simulink model "ePowertrain model"  (R2024b)
settings: Solver=VariableStepAuto  StartTime=0.0  StopTime=time  RelTol=1e-3
model workspace (MATLAB code in the model file):
  | RW = 0.254 ; % radius of vehicle (m)
  | GVM = 330 ; % gross vehicle mass (kg)
  | GVW = GVM*9.81 ; % gross vehicle weight (kg.m/s^2)
  | Crf = 0.015 ; % coeff of rolling resistance
  | slope_angle = 0 ; %slope angle in radian
  | Af = 1.1 ; %frontal Area (m^2)
  | Cd = 0.4 ; % coeff of drag
  | gear_ratio = 6 ;
  | trans_eff = 0.9; % transmission efficiency
  | motor_eff = 0.9; % motor efficiency
  | mc_eff = 0.95; % motor controller efficiency
  | Bv = 72 ; % battery voltage (V)
  | Cv = 3.6 ; % nominated cell votage (V)
  | Cc = 31 ; % cell capacity (Ah)
  | 
  | lap_distance = 0.787 ; % distance of one lap (km)
  | range = 20; % range of vehicle in single charge
  | time = 60 ; % time required to complete one lap
  | air_density = 1.225 ;
settings Model: Creator=chikr  LastModifiedBy=chikr

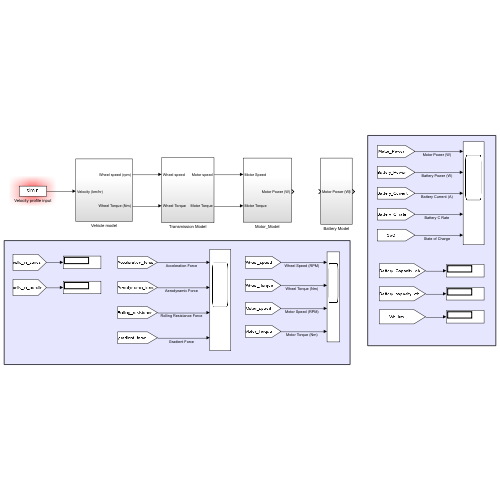
[thumbnail: Simulink's stored preview of the top-level diagram]
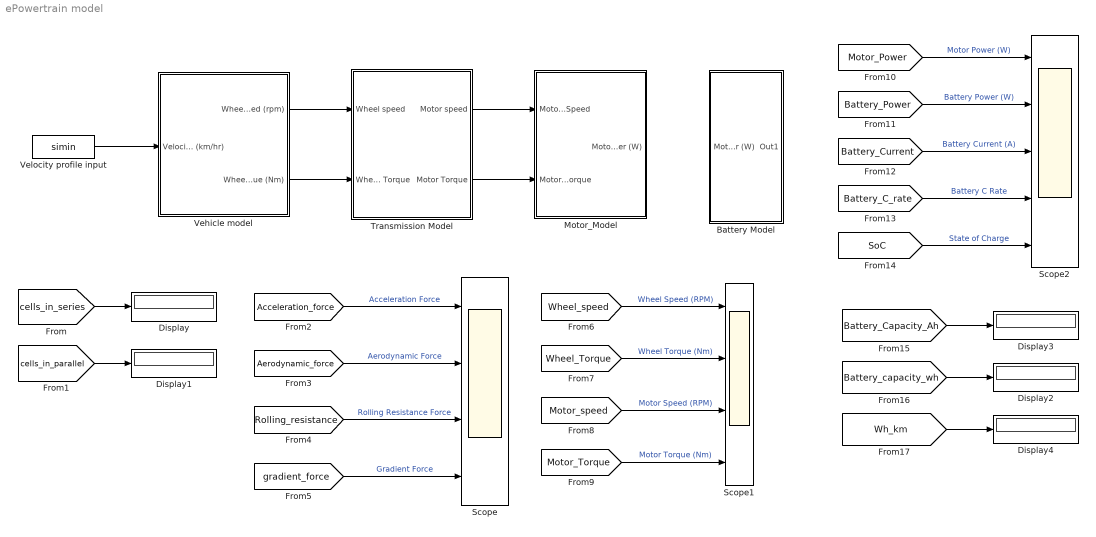
== system ePowertrain model ==
  Battery Model : Subsystem
  Display{,1..4} (5 alike) : Display
  Motor_Model : Subsystem
  Scope : Scope  NumInputPorts=4
  Scope1 : Scope  NumInputPorts=4
  Scope2 : Scope  NumInputPorts=5
  Transmission Model : Subsystem
  Vehicle model : Subsystem
  Velocity profile input : FromWorkspace  VariableName=simin
  wires:
  Velocity profile input/1 -> Vehicle model/1(Velocity (km/hr))
  Vehicle model/2(Wheel Torque (Nm)) -> Transmission Model/2(Wheel Torque)
  Vehicle model/1(Wheel speed (rpm)) -> Transmission Model/1(Wheel speed)
  Transmission Model/2(Motor Torque) -> Motor_Model/2(Motor Torque)
  Transmission Model/1(Motor speed) -> Motor_Model/1(Motor Speed)
  [cells_in_series] -> Display/1
  [cells_in_parallel] -> Display1/1
  [Acceleration_force] -> Scope/1  "Acceleration Force"
  [Aerodynamic_force] -> Scope/2  "Aerodynamic Force"
  [Rolling_resistance] -> Scope/3  "Rolling Resistance Force"
  [gradient_force] -> Scope/4  "Gradient Force"
  [Wheel_speed] -> Scope1/1  "Wheel Speed (RPM)"
  [Wheel_Torque] -> Scope1/2  "Wheel Torque (Nm)"
  [Motor_speed] -> Scope1/3  "Motor Speed (RPM)"
  [Motor_Torque] -> Scope1/4  "Motor Torque (Nm)"
  [Motor_Power] -> Scope2/1  "Motor Power (W)"
  [Battery_Current] -> Scope2/3  "Battery Current (A)"
  [Battery_Power] -> Scope2/2  "Battery Power (W)"
  [Battery_C_rate] -> Scope2/4  "Battery C Rate"
  [SoC] -> Scope2/5  "State of Charge"
  [Wh_km] -> Display4/1
  [Battery_capacity_wh] -> Display2/1
  [Battery_Capacity_Ah] -> Display3/1

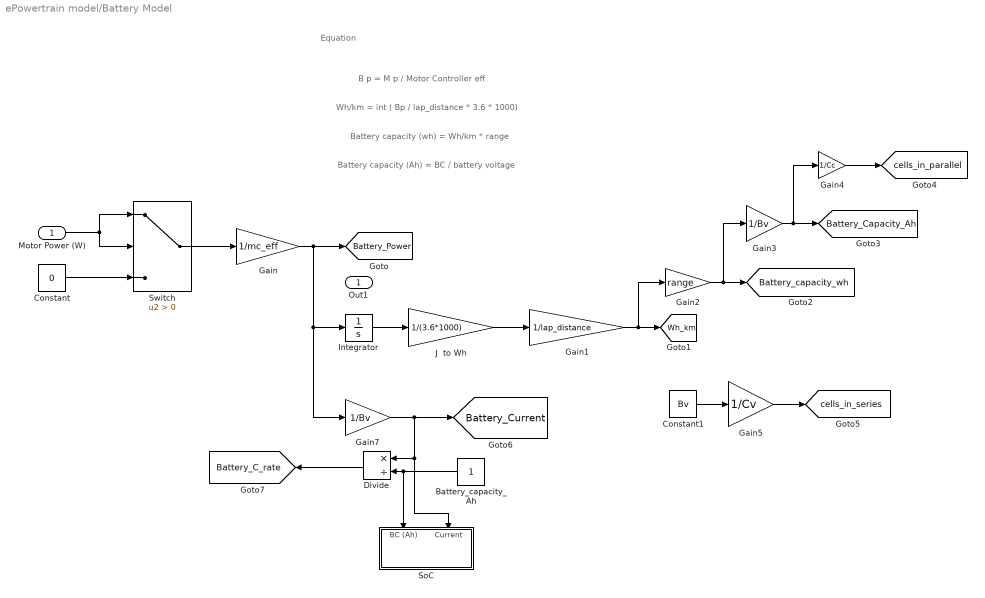
== system ePowertrain model/Battery Model ==
  note: Battery capacity (Ah) = BC / battery voltage
  note: Battery capacity (wh) = Wh/km * range
  note: Wh/km = int ( Bp / lap_distance * 3.6 * 1000)
  note: Equation
  note: B p = M p / Motor Controller eff
  Motor Power (W) : Inport
  Battery_capacity_Ah : Constant
  Constant : Constant  Value=0
  Constant1 : Constant  Value=Bv
  Divide : Product  Inputs=*/
  Gain : Gain  Gain=1/mc_eff
  Gain1 : Gain  Gain=1/lap_distance
  Gain2 : Gain  Gain=range
  Gain3 : Gain  Gain=1/Bv
  Gain4 : Gain  Gain=1/Cc
  Gain5 : Gain  Gain=1/Cv
  Gain7 : Gain  Gain=1/Bv
  Integrator : Integrator
  J  to Wh : Gain  Gain=1/(3.6*1000)
  SoC : Subsystem
      settings: PortSchema="{\"entries\":[{\"content\":{\"sides\":[{\"content\":{},\"type\":\"ConnectorPlacement.EquallySpacedRectSide\",\"uuid\":\"75e15061-75ea-40ab-85e0-9adabe2f895d\"},{\"content\":{\"side\":\"RIGHT\"},\"type\":\"ConnectorPlacement.EquallySpacedRectSide\",\"uuid\":\"53768e5b-e8ce-4d09-bbe5-28fa4e20151a\"},{\"content\":{\"connectorIds\":[\"In1\",\"In2\"],\"side\":\"TOP\"},\"type\":\"ConnectorPlacement.EquallySpacedRectSide\",\"uuid\":\"7db4e560-ff94-4941-b244-cacdfd66e211\"}]},\"type\":\"ConnectorPlacement.EquallySpacedConnector\",\"uuid\":\"b200b510-6a7e-48d6-8933-7bee46b324cd\"}],\"packageUris\":[\"http://schema.mathworks.com/mf0/Connector/R2020b\"],\"version\":\"1.0\"}"
  Switch : Switch  Criteria=u2 > Threshold  SaturateOnIntegerOverflow=off  InputSameDT=off
  Out1 : Outport
  tag scope: Battery_C_rate=global, Battery_Capacity_Ah=global, Battery_Current=global, Battery_Power=global, Battery_capacity_wh=global, Wh_km=global, cells_in_parallel=global, cells_in_series=global
  wires:
  Motor Power (W)/1 -> Switch/2, Switch/1
  Constant/1 -> Switch/3
  Switch/1 -> Gain/1
  Gain/1 -> Gain7/1, Integrator/1, [Battery_Power]
  Integrator/1 -> J  to Wh/1
  J  to Wh/1 -> Gain1/1
  Gain1/1 -> Gain2/1, [Wh_km]
  Gain2/1 -> Gain3/1, [Battery_capacity_wh]
  Gain3/1 -> Gain4/1, [Battery_Capacity_Ah]
  Gain4/1 -> [cells_in_parallel]
  Constant1/1 -> Gain5/1
  Gain5/1 -> [cells_in_series]
  Gain7/1 -> [Battery_Current], SoC/2(Current), Divide/1
  Battery_capacity_Ah/1 -> SoC/1(BC (Ah)), Divide/2
  Divide/1 -> [Battery_C_rate]

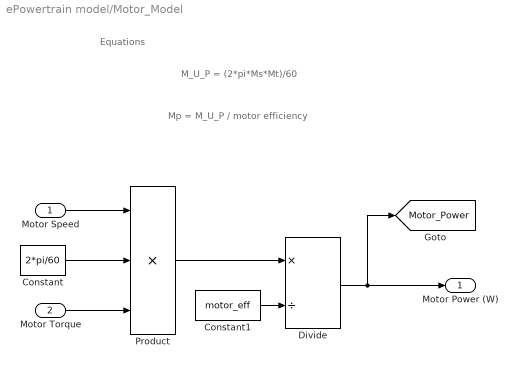
== system ePowertrain model/Motor_Model ==
  note: Equations
  note: Mp = M_U_P / motor efficiency
  note: M_U_P = (2*pi*Ms*Mt)/60
  Motor Speed : Inport
  Motor Torque : Inport  Port=2
  Constant : Constant  Value=2*pi/60
  Constant1 : Constant  Value=motor_eff
  Divide : Product  Inputs=*/
  Product : Product  Inputs=3
  Motor Power (W) : Outport
  tag scope: Motor_Power=global
  wires:
  Motor Speed/1 -> Product/1
  Motor Torque/1 -> Product/3
  Constant/1 -> Product/2
  Product/1 -> Divide/1
  Constant1/1 -> Divide/2
  Divide/1 -> [Motor_Power], Motor Power (W)/1

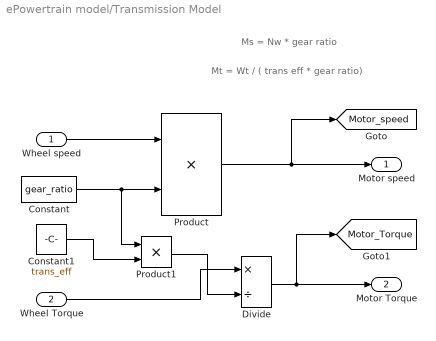
== system ePowertrain model/Transmission Model ==
  note: Mt = Wt / ( trans eff * gear ratio)
  note: Ms = Nw * gear ratio
  Wheel speed : Inport
  Wheel Torque : Inport  Port=2
  Constant : Constant  Value=gear_ratio
  Constant1 : Constant  Value=trans_eff
  Divide : Product  Inputs=*/
  Product : Product
  Product1 : Product
  Motor speed : Outport
  Motor Torque : Outport  Port=2
  tag scope: Motor_Torque=global, Motor_speed=global
  wires:
  Constant/1 -> Product1/1, Product/2
  Wheel speed/1 -> Product/1
  Product/1 -> [Motor_speed], Motor speed/1
  Constant1/1 -> Product1/2
  Wheel Torque/1 -> Divide/1
  Product1/1 -> Divide/2
  Divide/1 -> [Motor_Torque], Motor Torque/1

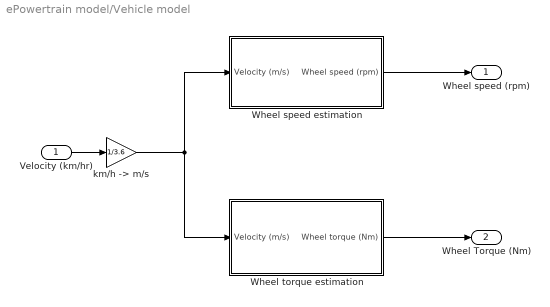
== system ePowertrain model/Vehicle model ==
  Velocity (km/hr) : Inport
  Wheel speed estimation : Subsystem
  Wheel torque estimation : Subsystem
  "km/h -> m/s" : Gain  Gain=1/3.6
  Wheel speed (rpm) : Outport
  Wheel Torque (Nm) : Outport  Port=2
  wires:
  Velocity (km/hr)/1 -> "km/h -> m/s"/1
  "km/h -> m/s"/1 -> Wheel torque estimation/1(Velocity (m/s)), Wheel speed estimation/1(Velocity (m/s))
  Wheel speed estimation/1(Wheel speed (rpm)) -> Wheel speed (rpm)/1
  Wheel torque estimation/1(Wheel torque (Nm)) -> Wheel Torque (Nm)/1

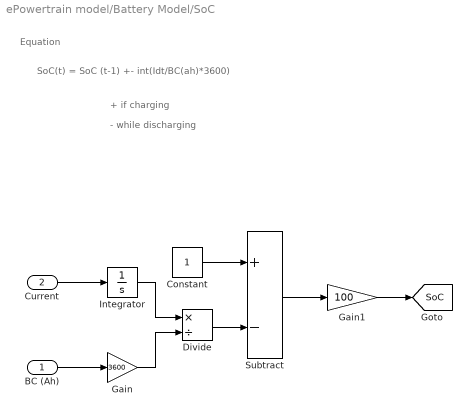
== system ePowertrain model/Battery Model/SoC ==
  note: Equation
  note: + if charging
  note: SoC(t) = SoC (t-1) +- int(Idt/BC(ah)*3600)
  note: - while discharging
  BC (Ah) : Inport
  Current : Inport  Port=2
  Constant : Constant
  Divide : Product  Inputs=*/
  Gain : Gain  Gain=3600
  Gain1 : Gain  Gain=100
  Integrator : Integrator
  Subtract : Sum  Inputs=+-
  tag scope: SoC=global
  wires:
  BC (Ah)/1 -> Gain/1
  Current/1 -> Integrator/1
  Gain/1 -> Divide/2
  Integrator/1 -> Divide/1
  Divide/1 -> Subtract/2
  Constant/1 -> Subtract/1
  Subtract/1 -> Gain1/1
  Gain1/1 -> [SoC]

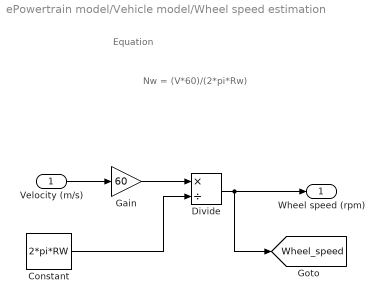
== system ePowertrain model/Vehicle model/Wheel speed estimation ==
  note: Equation
  note: Nw = (V*60)/(2*pi*Rw)
  Velocity (m/s) : Inport
  Constant : Constant  Value=2*pi*RW
  Divide : Product  Inputs=*/
  Gain : Gain  Gain=60
  Wheel speed (rpm) : Outport
  tag scope: Wheel_speed=global
  wires:
  Velocity (m/s)/1 -> Gain/1
  Constant/1 -> Divide/2
  Gain/1 -> Divide/1
  Divide/1 -> [Wheel_speed], Wheel speed (rpm)/1

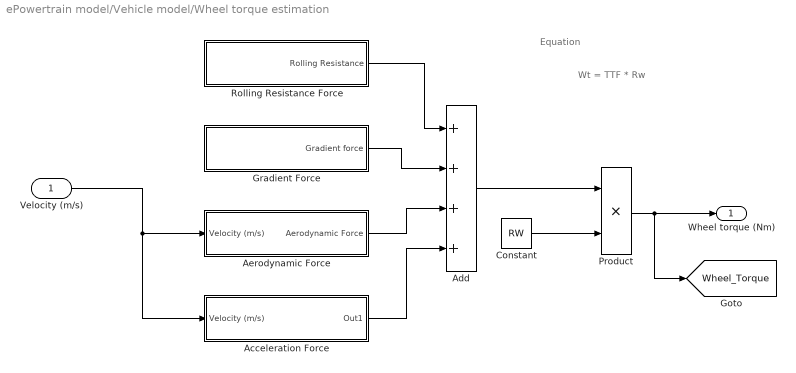
== system ePowertrain model/Vehicle model/Wheel torque estimation ==
  note: Equation
  note: Wt = TTF * Rw
  Velocity (m/s) : Inport
  Acceleration Force : Subsystem
  Add : Sum  Inputs=++++
  Aerodynamic Force : Subsystem
  Constant : Constant  Value=RW
  Gradient Force : Subsystem
  Product : Product
  Rolling Resistance Force : Subsystem
  Wheel torque (Nm) : Outport
  tag scope: Wheel_Torque=global
  wires:
  Velocity (m/s)/1 -> Aerodynamic Force/1(Velocity (m/s)), Acceleration Force/1(Velocity (m/s))
  Acceleration Force/1(Out1) -> Add/4
  Aerodynamic Force/1(Aerodynamic Force) -> Add/3
  Gradient Force/1(Gradient force) -> Add/2
  Rolling Resistance Force/1(Rolling Resistance) -> Add/1
  Constant/1 -> Product/2
  Add/1 -> Product/1
  Product/1 -> [Wheel_Torque], Wheel torque (Nm)/1

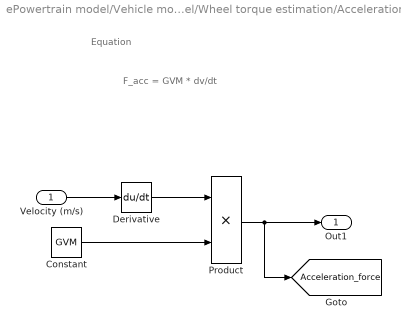
== system ePowertrain model/Vehicle model/Wheel torque estimation/Acceleration Force ==
  note: Equation
  note: F_acc = GVM * dv/dt
  Velocity (m/s) : Inport
  Constant : Constant  Value=GVM
  Derivative : Derivative
  Product : Product
  Out1 : Outport
  tag scope: Acceleration_force=global
  wires:
  Velocity (m/s)/1 -> Derivative/1
  Derivative/1 -> Product/1
  Constant/1 -> Product/2
  Product/1 -> [Acceleration_force], Out1/1

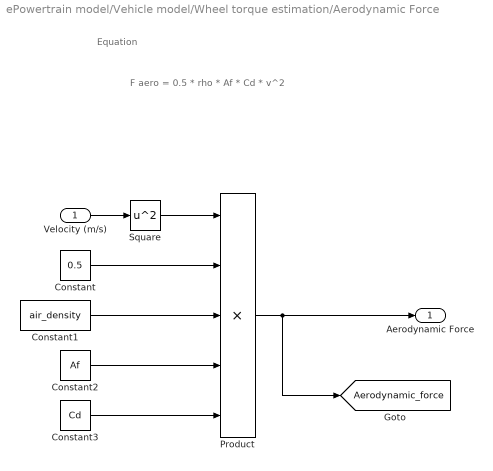
== system ePowertrain model/Vehicle model/Wheel torque estimation/Aerodynamic Force ==
  note: Equation
  note: F aero = 0.5 * rho * Af * Cd * v^2
  Velocity (m/s) : Inport
  Constant : Constant  Value=0.5
  Constant1 : Constant  Value=air_density
  Constant2 : Constant  Value=Af
  Constant3 : Constant  Value=Cd
  Product : Product  Inputs=5
  Square : Math  Operator=square
  Aerodynamic Force : Outport
  tag scope: Aerodynamic_force=global
  wires:
  Velocity (m/s)/1 -> Square/1
  Square/1 -> Product/1
  Constant/1 -> Product/2
  Constant1/1 -> Product/3
  Constant2/1 -> Product/4
  Constant3/1 -> Product/5
  Product/1 -> [Aerodynamic_force], Aerodynamic Force/1

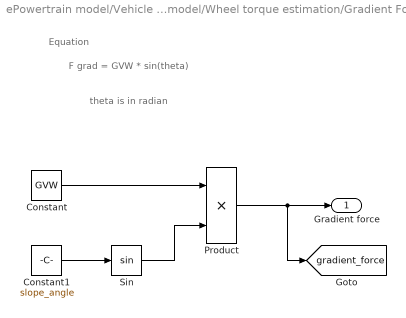
== system ePowertrain model/Vehicle model/Wheel torque estimation/Gradient Force ==
  note: Equation
  note: theta is in radian
  note: F grad = GVW * sin(theta)
  Constant : Constant  Value=GVW
  Constant1 : Constant  Value=slope_angle
  Product : Product
  Sin : Trigonometry
  Gradient force : Outport
  tag scope: gradient_force=global
  wires:
  Constant1/1 -> Sin/1
  Product/1 -> [gradient_force], Gradient force/1
  Constant/1 -> Product/1
  Sin/1 -> Product/2

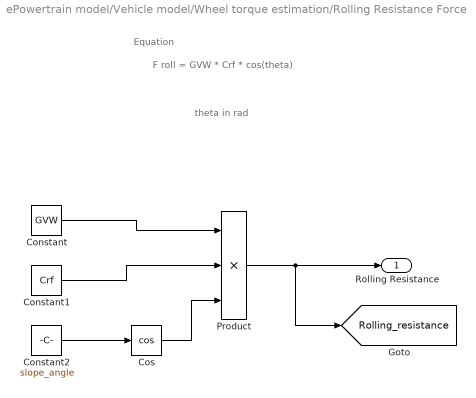
== system ePowertrain model/Vehicle model/Wheel torque estimation/Rolling Resistance Force ==
  note: Equation
  note: theta in rad
  note: F roll = GVW * Crf * cos(theta)
  Constant : Constant  Value=GVW
  Constant1 : Constant  Value=Crf
  Constant2 : Constant  Value=slope_angle
  Cos : Trigonometry  Operator=cos
  Product : Product  Inputs=3
  Rolling Resistance : Outport
  tag scope: Rolling_resistance=global
  wires:
  Constant2/1 -> Cos/1
  Cos/1 -> Product/3
  Constant1/1 -> Product/2
  Constant/1 -> Product/1
  Product/1 -> [Rolling_resistance], Rolling Resistance/1
